simulink library "thc"  (R2021b)
settings: Solver=VariableStepAuto  StartTime=0.0  StopTime=10.0  RelTol=1e-3
undefined symbols (not defined in the file or in its folder): ATHC_APTCQA_X_C, ATHC_APTCQB_X_C, ATHC_dAy_X_C, ATHC_Qeq_X_kmh, ATHC_VbaseC_X_C, ATHC_VbaseC_Y_W, ATHC_VbaseD_X_C, ATHC_VbaseH_X_C, FALSE, KTHC_ACMaxMinT_sec, KTHC_aDeice_K, KTHC_AGSDefLv_K, KTHC_AGSLv1_K, KTHC_AGSLv2_K, KTHC_AGSLv3_K, KTHC_AGSLv4_K, KTHC_AGSLv5_K, KTHC_AirIntUpdateT_sec, KTHC_APTCOneZoneMax_W, KTHC_APTCPeriod_cnt, KTHC_APTCPWMEN_flg, KTHC_APTCQMaxC_W, KTHC_APTCQminC_W, KTHC_APTCQminD_W, KTHC_APTCQminRe1_W, KTHC_APTCQminRe_W, KTHC_APTCQoffT_cnt, KTHC_APTCQonT_cnt, KTHC_APTCRiLeMaxDff_W, KTHC_APTCRiLeMinDff_W, KTHC_BatInTempDef_C, KTHC_bDeice_K, KTHC_CompMaxDeice_rpm, KTHC_CompMinDeice_rpm, KTHC_CompSotxvOp_K, KTHC_CompSotxvOpLow_rpm, KTHC_CompSpdmax_rpm, KTHC_CompSpdmaxBC1_rpm, KTHC_CompSpdmaxBC_rpm, KTHC_CompSpdmid1_rpm, KTHC_CompSpdmid2_rpm, KTHC_CompSpdmid3_rpm, KTHC_CompSpdmid_rpm, KTHC_CompSpdmin_rpm, KTHC_DAPTCQ1_W, KTHC_DAPTCQ2_W, KTHC_DAPTCQ3_W, KTHC_DcChSetTemp_C, KTHC_DehumidityEN_flg, KTHC_DeiceCycTime_K, KTHC_DriveLevelWPTCBAH1_W, KTHC_DriveLevelWPTCBAH2_W, KTHC_DriveLevelWPTCBAH3_W, KTHC_DriveLevelWPTCBAH4_W, KTHC_DriveT1MinBAH_C, KTHC_DriveT2MaxBAH_C, KTHC_DriveT2MinBAH_C, KTHC_DriveT3MaxBAH_C, KTHC_DriveT3MinBAH_C, KTHC_DriveT4MaxBAH_C ... (+372)
libraries: simulink x140
(part 10 of 10)

== stateflow chart thc/THC/ThermalControl/THCM_Conctrl/APTC/APTCPWMControl1/Chart ==
  state APTC
    en:
    Wout=Win;
    du:
    Wout=Win;
  state APTCPWM
    (default) -> (junction 5) : {Tcnt=0;OnT=0;OffT=0;}
    APTCPWM -> (junction 5) [order 1]
    (junction 5) -> (junction 7) [order 1] : [Win==0]{Wout=0;}
    (junction 5) -> (junction 9) [order 2]
    (junction 7) -> (junction 11)
    (junction 9) -> (junction 11) [order 1] : [Win>Wmin]{Wout=Win;}
    (junction 9) -> (junction 54) [order 2]
    (junction 11) -> (junction 56)
    (junction 54) -> (junction 56) [order 1] : [Wout>Wmin]{Tcnt=0;Wout=0;....
        | OnT=Tp*Win/Wmin;OffT=Tp-OnT;}
    (junction 54) -> (junction 13) [order 2]
    (junction 56) -> (junction 15)
    (junction 13) -> (junction 15) [order 1] : [Wout>0&&Tcnt>=OnT]
        | {Tcnt=0;Wout=0;}
    (junction 13) -> (junction 17) [order 2]
    (junction 15) -> (junction 19)
    (junction 17) -> (junction 19) [order 1] : [Wout==0&&Tcnt>=OffT]
        | {Tcnt=0;Wout=Wmin;....
        | OnT=Tp*Win/Wmin;OffT=Tp-OnT;}
    (junction 17) -> (junction 26) [order 2]
    (junction 19) -> (junction 28)
    (junction 26) -> (junction 28)
    (junction 28) -> (junction 31) [order 2] : {Tcnt=Tcnt+1;}
    (junction 28) -> (junction 33) [order 1] : [Tcnt>Tp||(OnT==0&&OffT==0)]
        | {Tcnt=0;OnT=0;OffT=0;}
  (default) -> (junction 50)
  (junction 50) -> APTC [order 1] : [!KTHC_APTCPWMEN_flg]
  (junction 50) -> APTCPWM [order 2]
  APTCPWM -> APTC [order 1] : [!KTHC_APTCPWMEN_flg]
  APTC -> APTCPWM : [KTHC_APTCPWMEN_flg]
  data: OnT local uint16; OffT local uint16; Tcnt local uint16; Win input; Wout output uint16; Tp input uint16; Wmin input; KTHC_APTCPWMEN_flg input

== stateflow chart thc/THC/ThermalControl/THCM_Conctrl/APTC/APTCPWMControl2/Chart ==
  state APTC
    en:
    Wout=Win;
    du:
    Wout=Win;
  state APTCPWM
    (default) -> (junction 5) : {Tcnt=0;OnT=0;OffT=0;}
    APTCPWM -> (junction 5) [order 1]
    (junction 5) -> (junction 7) [order 1] : [Win==0]{Wout=0;}
    (junction 5) -> (junction 9) [order 2]
    (junction 7) -> (junction 11)
    (junction 9) -> (junction 11) [order 1] : [Win>Wmin]{Wout=Win;}
    (junction 9) -> (junction 54) [order 2]
    (junction 11) -> (junction 56)
    (junction 54) -> (junction 56) [order 1] : [Wout>Wmin]{Tcnt=0;Wout=0;....
        | OnT=Tp*Win/Wmin;OffT=Tp-OnT;}
    (junction 54) -> (junction 13) [order 2]
    (junction 56) -> (junction 15)
    (junction 13) -> (junction 15) [order 1] : [Wout>0&&Tcnt>=OnT]
        | {Tcnt=0;Wout=0;}
    (junction 13) -> (junction 17) [order 2]
    (junction 15) -> (junction 19)
    (junction 17) -> (junction 19) [order 1] : [Wout==0&&Tcnt>=OffT]
        | {Tcnt=0;Wout=Wmin;....
        | OnT=Tp*Win/Wmin;OffT=Tp-OnT;}
    (junction 17) -> (junction 26) [order 2]
    (junction 19) -> (junction 28)
    (junction 26) -> (junction 28)
    (junction 28) -> (junction 31) [order 2] : {Tcnt=Tcnt+1;}
    (junction 28) -> (junction 33) [order 1] : [Tcnt>Tp||(OnT==0&&OffT==0)]
        | {Tcnt=0;OnT=0;OffT=0;}
  (default) -> (junction 50)
  (junction 50) -> APTC [order 1] : [!KTHC_APTCPWMEN_flg]
  (junction 50) -> APTCPWM [order 2]
  APTCPWM -> APTC [order 1] : [!KTHC_APTCPWMEN_flg]
  APTC -> APTCPWM : [KTHC_APTCPWMEN_flg]
  data: OnT local uint16; OffT local uint16; Tcnt local uint16; Win input; Wout output uint16; Tp input uint16; Wmin input; KTHC_APTCPWMEN_flg input

== stateflow chart thc/THC/ThermalControl/THCM_Conctrl/BlowerCtrl/Chart ==
  state VGainCal
    (default) -> (junction 7)
    (junction 7) -> (junction 8) [order 1] : [VFull]
    (junction 7) -> (junction 10) [order 2] : {VGain=KTHC_VBRearClosed_K;}
    (junction 8) -> (junction 12) : {VGain=1;}
    (junction 10) -> (junction 12)
    (junction 12) -> (junction 15)
    VGainCal -> (junction 17) [order 1] : [VFull&&VGain<1]
    (junction 17) -> (junction 19) [order 1] : [VGain+KTHC_VGainStep_K<1]
    (junction 17) -> (junction 25) [order 2] : {VGain=1;}
    (junction 19) -> (junction 23) : {VGain=VGain+KTHC_VGainStep_K;}
    (junction 25) -> (junction 23)
    (junction 23) -> (junction 15)
    (junction 15) -> (junction 36)
    VGainCal -> (junction 21) [order 2] : [!VFull&&VGain>KTHC_VBRearClosed_K]
    (junction 21) -> (junction 28) [order 1] : [VGain-KTHC_VGainStep_K>KTHC_VBRearClosed_K]
    (junction 21) -> (junction 30) [order 2] : {VGain=KTHC_VBRearClosed_K;}
    (junction 28) -> (junction 32) : {VGain=VGain-KTHC_VGainStep_K;}
    (junction 30) -> (junction 32)
    (junction 32) -> (junction 36)
  data: VGain output single; VFull input boolean; KTHC_VBRearClosed_K input; KTHC_VGainStep_K input

== stateflow chart thc/THC/ThermalControl/THCM_Conctrl/Subsystem3/Chart ==
  state FWVSWReqDet [parallel]
    settings: executionOrder=2
    state StandBy
    (default) -> FWVSWReqDet.StandBy : {FWVSWReq=false;}
    FWVSWReqDet.StandBy -> FWVSWReqDet.StandBy : [AllStopReq]{FWVSWReq=true;}
  state EWP12Stop [parallel]
    settings: executionOrder=1
    state SpeedBalance
      state Stop
        en:EWP12Stop=true;
      state Wait
      (default) -> EWP12Stop.SpeedBalance.Stop
      EWP12Stop.SpeedBalance.Wait -> EWP12Stop.SpeedBalance.Stop : [after(EWPStopT,tick)]
    state NotBalance
      en:EWP12Stop=false;
    (default) -> EWP12Stop.SpeedBalance
    EWP12Stop.SpeedBalance -> EWP12Stop.NotBalance : [EWP1!=EWP2||....
        | hasChanged(EWP1)||....
        | hasChanged(EWP2)]
    EWP12Stop.NotBalance -> EWP12Stop.SpeedBalance.Wait : [EWP1==EWP2]
  state ValveControl [parallel]
    settings: executionOrder=4
    state StandBy
      en:
      TWVKeep=false;
      FWVKeep=false;
      EWPKeep=false;
      ex:
      TWVKeep=true;
      FWVKeep=true;
    state WaitEWPPartBallance
    state WaitEWPallStop
      ex:FWVSWReq=false;
      FWVKeep=false;
    state EWPKeep
      en:EWPKeep=true;
      TWVKeep=false;
      ex:EWPKeep=false;
    (default) -> ValveControl.StandBy
    ValveControl.StandBy -> WaitEWPPartBallance [order 2] : [PartStopReq]
    ValveControl.StandBy -> (junction 42) [order 1]
    WaitEWPPartBallance -> (junction 42) [order 2]
    (junction 42) -> WaitEWPallStop : [FWVSWReq]
    (junction 97) -> ValveControl.StandBy [order 2]
    WaitEWPPartBallance -> EWPKeep [order 1] : [EWP12Stop]
    (junction 97) -> WaitEWPallStop [order 1] : [FWVSWReq]
    EWPKeep -> (junction 97) : [after(ValueSWT,tick)]
    WaitEWPallStop -> EWPKeep : [EWPAllStop]
  state EWPAllStop [parallel]
    settings: executionOrder=3
    state SpeedBalance
      state Stop
        en:EWPAllStop=true;
      state Wait
      (default) -> EWPAllStop.SpeedBalance.Stop
      EWPAllStop.SpeedBalance.Wait -> EWPAllStop.SpeedBalance.Stop : [after(EWPStopT,tick)]
    state NotBalance
      en:EWPAllStop=false;
    (default) -> EWPAllStop.SpeedBalance
    EWPAllStop.SpeedBalance -> EWPAllStop.NotBalance : [EWP1!=EWP2||....
        | EWP2!=EWP3]
    EWPAllStop.NotBalance -> EWPAllStop.SpeedBalance.Wait : [EWP1==EWP2&&....
        | EWP2==EWP3]
  data: TWVKeep output boolean; FWVKeep output boolean; PartStopReq input boolean; AllStopReq input boolean; EWP1 input uint8; EWP2 input uint8; EWP3 input uint8; EWP12Stop local boolean; EWPAllStop local boolean; EWPStopT input uint8; ValueSWT input uint8; EWPKeep output boolean; FWVSWReq local boolean

== stateflow chart thc/THC/ThermalControl/AC1/Chart ==
  state Sync [parallel]
    settings: executionOrder=1
    state WaitForIVI
    state Release
    state Press
      state Wait
      state Over10sec
        en:ACForceOFF=!ACForceOFF;
      (default) -> Wait
      Wait -> Over10sec : [after(100,tick)]
    (default) -> WaitForIVI : {CCU_SyncSts=EEP_CCUSyncSts;ACForceOFF=EEP_ACForceOFF;}
    WaitForIVI -> Sync.Release : [VINP_CANMsgValidIVI2_flg]
    Sync.Release -> Sync.Release [order 3] : [SyncCancel]
        | {CCU_SyncSts=false;}
    Sync.Release -> Sync.Release [order 2] : [hasChanged(sigSetTempZon2Req_CMD)&&....
        | (sigSetTempZon2Req_CMD) != (sigSetTempZon1Req_CMD)]
        | {CCU_SyncSts=false;}
    Sync.Release -> Sync.Press [order 1] : [FCP_FrEvt_BtnSyncReq]
        | {CCU_SyncSts=!CCU_SyncSts;}
    Sync.Press -> Sync.Release [order 1] : [!FCP_FrEvt_BtnSyncReq]
    Sync.Press -> Sync.Press [order 2] : [SyncCancel]
        | {CCU_SyncSts=false;}
    Sync.Press -> Sync.Press [order 3] : [hasChanged(sigSetTempZon2Req_CMD)&&....
        | (sigSetTempZon2Req_CMD) != (sigSetTempZon1Req_CMD)]
        | {CCU_SyncSts=false;}
  state Recycle [parallel]
    settings: executionOrder=15
    state Manual
      state Outter
        en:sigRecircSt=false;
        state ACOFF
          en:FD_RecyAuto_Cmd=0;
        state ACON
          en:FD_RecyAuto_Cmd=4;
        (default) -> (junction 1044)
        (junction 1044) -> ACOFF [order 1] : [!CCU_ACLampSts&&....
            | (CabinMode==11&&....
            | ACSubMode==1)]
        (junction 1044) -> ACON [order 2]
        ACON -> ACOFF : [!CCU_ACLampSts&&....
            | (CabinMode==11&&ACSubMode==1)]
        ACOFF -> ACON : [CCU_ACLampSts||....
            | (CabinMode!=11||ACSubMode!=1)]
      state Inner
        en:sigRecircSt=true;
        FD_RecyAuto_Cmd=0;
      (default) -> (junction 920)
      (junction 920) -> (junction 922) [order 1] : [EEP_sigRecircSt]
      (junction 920) -> Outter [order 2]
      (junction 922) -> Inner
      Inner -> Outter [order 2] : eDefogRecycle
      Outter -> Inner : eRecycleBtn
      Inner -> Outter [order 1] : eRecycleBtn
      (junction 839) -> Outter [order 1] : [sigRecircSt]
      (junction 839) -> Inner [order 2]
    state Auto
      state SetLowT
        en:sigRecircSt=false;FD_RecyAuto_Cmd=4;
      state Normal
        state AutoInner
          en:
          sigRecircSt=true;
          note: 2 min
          state Refresh
            en:
            FD_RecyAuto_Cmd=4;
          state Hold
            en:
            FD_RecyAuto_Cmd=0;
          (default) -> Hold
          Refresh -> Hold : [after(KTHC_RecyChange_min*600,tick)]
          Hold -> Refresh : [KTHC_RefreshEN_flg&&...
              | after(KTHC_RecyHold_min*600,tick)]
        note: 30 min
        state AutoOutter
          en:sigRecircSt=false;
          state Dehumidity
            en:FD_RecyAuto_Cmd=KTHC_RecyOutterD_enum;
          state Normal
            state LV5
              en:FD_RecyAuto_Cmd=4;
            state LV4
              en:FD_RecyAuto_Cmd=3;
            state LV3
              en:FD_RecyAuto_Cmd=2;
            state LV2
              en:FD_RecyAuto_Cmd=1;
            (junction 713) -> LV5 [order 1] : [Tamb>KTHC_T4Mmaxamb_C]
            (junction 713) -> (junction 719) [order 2]
            LV5 -> LV4 : [Tamb<KTHC_T5Mminamb_C]
            LV4 -> LV5 [order 1] : [Tamb>KTHC_T4Mmaxamb_C]
            (junction 719) -> LV4 [order 1] : [Tamb>KTHC_T3Mmaxamb_C]
            (junction 719) -> (junction 725) [order 2]
            LV4 -> LV3 [order 2] : [Tamb<KTHC_T4Mminamb_C]
            LV3 -> LV4 [order 1] : [Tamb>KTHC_T3Mmaxamb_C]
            (junction 725) -> LV3 [order 1] : [Tamb>KTHC_T2Mmaxamb_C]
            (junction 725) -> (junction 730) [order 2]
            LV3 -> LV2 [order 2] : [Tamb<KTHC_T3Mminamb_C]
            LV2 -> LV3 : [Tamb>KTHC_T2Mmaxamb_C]
            (junction 730) -> LV2
          (default) -> (junction 1030)
          (junction 1030) -> Dehumidity [order 1] : [CabinMode<7]
          (junction 1030) -> (junction 1034) [order 2]
          Dehumidity -> (junction 1034) : [CabinMode>=7]
          (junction 1034) -> (junction 713)
          Recycle.Auto.Normal.AutoOutter.Normal -> Dehumidity : [CabinMode<7]
        (default) -> (junction 752)
        (junction 752) -> AutoInner [order 1] : [CabinMode==3||....
            | CabinMode==6||....
            | (CabinMode==11&&....
            | ACSubMode==1)]
        (junction 752) -> (junction 754) [order 2]
        AutoInner -> (junction 754) : [CabinMode!=3&&....
            | CabinMode!=6&&....
            | (CabinMode!=11||....
            | ACSubMode!=1)]
        (junction 754) -> AutoOutter
        AutoOutter -> AutoInner : [CabinMode==3||CabinMode==6||....
            | (CabinMode==11&&ACSubMode==1)]
      (default) -> (junction 1010)
      (junction 1010) -> (junction 1014) [order 1]
      (junction 1014) -> SetLowT : [CabinMode==3&&(ACSubMode==2||ACSubMode==6||ACSubMode==7)....
          | &&SetTempZon1St_CMD==170&&Tamb<KTHC_Trecymin_C]
      SetLowT -> Recycle.Auto.Normal : [CabinMode!=3||(ACSubMode!=2&&ACSubMode!=6&&ACSubMode!=7)||....
          | SetTempZon1St_CMD>170||Tamb>=KTHC_Trecymin_C]
      (junction 1010) -> Recycle.Auto.Normal [order 2]
      Recycle.Auto.Normal -> (junction 1014)
    (default) -> (junction 914)
    (junction 914) -> Recycle.Manual [order 1] : [EEP_ACModeMem!=2||!EEP_RecAutoFlg]
        | {RecAutoFlg=EEP_RecAutoFlg;}
    (junction 914) -> (junction 917) [order 2]
    Recycle.Auto -> (junction 839) [order 3] : eRecycleBtn
    Recycle.Auto -> Outter [order 2] : [!CCU_AutoLampSts&&!RecAutoFlg&&!sigRecircSt]
    Recycle.Auto -> Outter [order 1] : eDefogRecycle
    Recycle.Auto -> Inner [order 4] : [!CCU_AutoLampSts&&!RecAutoFlg]
    Recycle.Manual -> Recycle.Auto [order 2] : eACMaxRec
    Recycle.Manual -> Recycle.Auto [order 1] : [CCU_AutoLampSts&&RecAutoFlg]
    (junction 917) -> Recycle.Auto
  state RecycleSW [parallel]
    settings: executionOrder=16
    state Release
    state Press
      en:Recycle.eRecycleBtn;
      RecAutoFlg=false;
    (default) -> RecycleSW.Release
    RecycleSW.Release -> RecycleSW.Press : [sigRecircReq]
    RecycleSW.Press -> RecycleSW.Release : [!sigRecircReq]
  state PETMODE [parallel]
    settings: executionOrder=18
    state OFF
      en:PET=false;
    state ON
      en:PET=true;
    (default) -> PETMODE.OFF
    PETMODE.OFF -> PETMODE.ON : [(PwrSta>0&&PwrSta<=3&&(OFF_AC_MODE==1||OFF_AC_MODE==2||VINP_RemoteAutoReq_flg))||(ForceAuto&&PwrSta>3)]
    PETMODE.ON -> PETMODE.OFF : [(PwrSta==0||PwrSta>3||(OFF_AC_MODE!=1&&OFF_AC_MODE!=2&&!VINP_RemoteAutoReq_flg))&&(!ForceAuto||PwrSta<=3)]
  state ACBtn [parallel]
    settings: executionOrder=2
    state Initial
    state Release
    state Press
      en:AC.ACMode.eACBtn;
      WaterFill.eACBtn;
    (default) -> ACBtn.Initial
    ACBtn.Initial -> (junction 899) [order 2]
    (junction 899) -> ACBtn.Press
    ACBtn.Initial -> ACBtn.Release [order 1] : [EEP_ACModeMem!=1]
    ACBtn.Press -> ACBtn.Release : [!FCP_FrEvt_BtnACReq]
    ACBtn.Release -> ACBtn.Press : [FCP_FrEvt_BtnACReq]
  state ACAutoBtn [parallel]
    settings: executionOrder=3
    state Initial
    state Release
    state Press
      en:
      WaterFill.eACAutoBtn;
      RecAutoFlg=true;
    (default) -> ACAutoBtn.Initial
    ACAutoBtn.Initial -> (junction 904) [order 2] : {AC.ACMode.eACAutoBtn;}
    (junction 904) -> ACAutoBtn.Release
    ACAutoBtn.Initial -> ACAutoBtn.Release [order 1] : [EEP_ACModeMem!=2]
    ACAutoBtn.Release -> (junction 700) : [FCP_FrEvt_BtnAutoReq]
    (junction 700) -> ACAutoBtn.Press [order 1] : [CCU_AutoLampSts]{AC.ACMode.eAutoexit;}
    (junction 700) -> (junction 702) [order 2]
    (junction 702) -> ACAutoBtn.Press : {AC.ACMode.eACAutoBtn;}
    ACAutoBtn.Press -> ACAutoBtn.Release : [!FCP_FrEvt_BtnAutoReq]
  state ACMaxBtn [parallel]
    settings: executionOrder=4
    state Release
    state Press
      en:AC.ACMode.eACMaxBtn;
    (default) -> ACMaxBtn.Release
    ACMaxBtn.Release -> ACMaxBtn.Press : [FCP_FrEvt_BtnACMaxReq]
    ACMaxBtn.Press -> ACMaxBtn.Release : [!FCP_FrEvt_BtnACMaxReq]
  state ScreenBtn [parallel]
    settings: executionOrder=8
    state Release
    state Press
      en:AC.ACMode.eAutoexit;
    (default) -> ScreenBtn.Release
    ScreenBtn.Press -> ScreenBtn.Release : [!sigScreenReq]
    ScreenBtn.Release -> (junction 1060) : [sigScreenReq]{fdefog=false;}
    (junction 1060) -> ScreenBtn.Press [order 1] : [!Face&&!Foot&&Frost]
    (junction 1060) -> (junction 1061) [order 2]
    (junction 1061) -> ScreenBtn.Press : {Frost=!Frost;}
  state FaceBtn [parallel]
    settings: executionOrder=5
    state Press
      en:AC.ACMode.eAutoexit;
    state Release
    (default) -> FaceBtn.Release : {Face=EEP_Face;}
    FaceBtn.Press -> FaceBtn.Release : [!sigFaceReq]
    FaceBtn.Release -> (junction 183) : [sigFaceReq]{fdefog=false;}
    (junction 183) -> FaceBtn.Press [order 1] : [Face&&!Foot&&!Frost]
    (junction 183) -> (junction 185) [order 2]
    (junction 185) -> FaceBtn.Press : {Face=!Face;}
  state FootBtn [parallel]
    settings: executionOrder=6
    state Release
    state Press
      en:AC.ACMode.eAutoexit;
    (default) -> FootBtn.Release : {Foot=EEP_Foot;}
    FootBtn.Press -> FootBtn.Release : [!sigFootReq]
    FootBtn.Release -> (junction 189) : [sigFootReq]{fdefog=false;}
    (junction 189) -> FootBtn.Press [order 1] : [!Face&&Foot&&!Frost]
    (junction 189) -> (junction 197) [order 2]
    (junction 197) -> FootBtn.Press : {Foot=!Foot;}
  state Frost [parallel]
    settings: executionOrder=7
    state Press
      en:AC.ACMode.eAutoexit;
      ACModeMem=1;
    state Release
    (default) -> Frost.Release : {Frost=EEP_Frost;FaceM=EEP_FaceM;FootM=EEP_FootM;fdefog=EEP_fdefog;}
    Frost.Press -> Frost.Release : [!sigFrostReq]
    Frost.Release -> (junction 206) : [sigFrostReq]
    (junction 206) -> (junction 1208) [order 1] : [KTHC_ScreenUniq_flg&&!fdefog]
    (junction 206) -> (junction 1204) [order 2]
    (junction 1208) -> (junction 1206)
    (junction 1204) -> (junction 1206) [order 1] : [!KTHC_ScreenUniq_flg&&!Frost]
    (junction 1206) -> Frost.Press : {Frost=true;FaceM=Face;FootM=Foot;....
        | Face=false;Foot=false;fdefog=true;....
        | Recycle.eDefogRecycle;RecAutoFlg=false;}
    (junction 1204) -> (junction 200) [order 2]
    (junction 200) -> (junction 1212) [order 1] : [!Face&&!Foot]{Face=FaceM;Foot=FootM;fdefog=false;}
    (junction 1212) -> Frost.Press [order 1] : [!FaceM&&!FootM]{Frost=true;}
    (junction 200) -> (junction 769) [order 2]
    (junction 1212) -> (junction 1214) [order 2]
    (junction 1214) -> Frost.Press : {Frost=false;}
    (junction 769) -> Frost.Press : {Frost=false;fdefog=false;}
  state HMIWindDir [parallel]
    settings: executionOrder=9
    state StandBy
      ex:fdefog=0;
    (default) -> StandBy
    StandBy -> (junction 1100) [order 1] : [WindDirP]
    (junction 1100) -> (junction 1129) [order 1] : [sigWindDirZon1St==6]
        | {sigWindDirZon1StTemp=0;}
    (junction 1100) -> (junction 1127) [order 2]
    (junction 1129) -> (junction 1130)
    (junction 1127) -> (junction 1130) : {sigWindDirZon1StTemp=sigWindDirZon1St+1;}
    (junction 1130) -> (junction 1136)
    StandBy -> (junction 1133) [order 2] : [WindDirM]
    (junction 1133) -> (junction 1136) [order 1] : [sigWindDirZon1St==0]
        | {sigWindDirZon1StTemp=6;}
    (junction 1133) -> (junction 1138) [order 2]
    (junction 1136) -> (junction 1140)
    (junction 1138) -> (junction 1140) : {sigWindDirZon1StTemp=sigWindDirZon1St-1;}
    (junction 1140) -> (junction 1153)
    (junction 1153) -> StandBy [order 1] : [sigWindDirZon1StTemp==0]{Face=1;Foot=0;Frost=0;}
    (junction 1153) -> (junction 1156) [order 2]
    (junction 1156) -> StandBy [order 1] : [sigWindDirZon1StTemp==1]{Face=1;Foot=1;Frost=0;}
    (junction 1156) -> (junction 1159) [order 2]
    (junction 1159) -> StandBy [order 1] : [sigWindDirZon1StTemp==2]{Face=0;Foot=1;Frost=0;}
    (junction 1159) -> (junction 1162) [order 2]
    (junction 1162) -> StandBy [order 1] : [sigWindDirZon1StTemp==3]{Face=0;Foot=1;Frost=1;}
    (junction 1162) -> (junction 1165) [order 2]
    (junction 1165) -> StandBy [order 1] : [sigWindDirZon1StTemp==4]{Face=0;Foot=0;Frost=1;}
    (junction 1165) -> (junction 1168) [order 2]
    (junction 1168) -> StandBy [order 1] : [sigWindDirZon1StTemp==5]{Face=1;Foot=0;Frost=1;}
    (junction 1168) -> (junction 1171) [order 2]
    (junction 1171) -> StandBy : {Face=1;Foot=1;Frost=1;}
  state AC [parallel]
    settings: executionOrder=17
    state ACMode
      state ON
        state Max
          en:
          CCU_ACLampSts=true;
          CCU_AutoLampSts=false;
          CCU_ACMaxLampSts=true;
          sigAirIntenZon1St=9;
          CCU_SyncSts=true;
          Recycle.eACMaxRec;
          RecAutoFlg=true;
          state WaitMinT
          state WaitFinish
          (default) -> WaitMinT
          WaitMinT -> WaitFinish : [after(KTHC_ACMaxMinT_sec*10,tick)]
        state Manual
          en:
          CCU_ACLampSts=true;CCU_AutoLampSts=false;
          CCU_ACMaxLampSts=false;ACModeMem=1;
          RecAutoFlg=false;
          ACModeMem = 1;
          state Normal
            en:
            sigAirIntenZon1St=AirIntenZone1M;
            du:
            sigAirIntenZon1St=AirIntenZone1M;
          state DeFog
            en:
            sigAirIntenZon1St=9;
            ex:
            fdefog=false;
          (default) -> (junction 779)
          (junction 779) -> DeFog [order 2]
          (junction 779) -> AC.ACMode.ON.Manual.Normal [order 1] : [!fdefog]
          DeFog -> AC.ACMode.ON.Manual.Normal : [!fdefog]
          AC.ACMode.ON.Manual.Normal -> DeFog : [fdefog]
        state Auto
          en:
          CCU_ACLampSts=true;
          CCU_AutoLampSts=true;
          CCU_ACMaxLampSts=false;
          ACModeMem=2;
        WaitFinish -> (junction 851) : [MaxFinish||....
            | !CCU_SyncSts]
        Max -> AC.ACMode.ON.Manual [order 2] : eACMaxexit
        AC.ACMode.ON.Manual -> Max : eACMaxBtn
        Max -> (junction 850) [order 1] : eACMaxBtn
        AC.ACMode.ON.Auto -> Max [order 1] : eACMaxBtn
        (junction 850) -> (junction 851)
        (junction 851) -> (junction 49)
        (junction 49) -> AC.ACMode.ON.Manual [order 2]
        (junction 49) -> AC.ACMode.ON.Auto [order 1] : [ACModeMem==2]
        AC.ACMode.ON.Auto -> AC.ACMode.ON.Manual [order 2] : eAutoexit
        AC.ACMode.ON -> AC.ACMode.ON.Auto [order 1] : eACAutoBtn
        (default) -> (junction 943)
        (junction 943) -> AC.ACMode.ON.Manual [order 2]
        (junction 943) -> AC.ACMode.ON.Auto [order 1] : [ACModeMem == 2]
      state OFF
        en:
        CCU_ACLampSts=false;
        CCU_AutoLampSts=false;
        CCU_ACMaxLampSts=false;
        ACModeMem=0;
        sigAirIntenZon1St=AirIntenZone1M;
        du:
        sigAirIntenZon1St=AirIntenZone1M;
      (default) -> AC.ACMode.OFF
      AC.ACMode.OFF -> (junction 669) [order 4] : eACMaxBtn{ACModeMem=1;}
      (junction 669) -> Max [order 1] : [AirIntenZone1M!=1]
      (junction 669) -> (junction 671) [order 2]
      (junction 671) -> Max : {AirIntenZone1M=2;}
      AC.ACMode.ON -> AC.ACMode.OFF [order 1] : eACBtn
      AC.ACMode.OFF -> (junction 832) [order 2] : eACBtn
      (junction 832) -> (junction 833)
      AC.ACMode.OFF -> (junction 833) [order 1] : [fdefog]
      (junction 833) -> (junction 674)
      (junction 674) -> AC.ACMode.ON.Manual [order 1] : [AirIntenZone1M!=1]
      (junction 674) -> (junction 677) [order 2]
      (junction 677) -> AC.ACMode.ON.Manual : {AirIntenZone1M=2;}
      AC.ACMode.ON -> AC.ACMode.OFF [order 2] : [sigAirIntenZon1Req==1]
      (junction 683) -> AC.ACMode.ON.Auto [order 1] : [AirIntenZone1M!=1]
      AC.ACMode.OFF -> (junction 683) [order 3] : eACAutoBtn
      (junction 683) -> (junction 680) [order 2]
      (junction 680) -> AC.ACMode.ON.Auto : {AirIntenZone1M=2;}
      (junction 948) -> AC.ACMode.OFF [order 1] : [ACModeMem == 0]
      (junction 948) -> AC.ACMode.ON [order 2]
      (junction 947) -> (junction 948)
    state PET
      en:
      CCU_ACLampSts=true;
      CCU_AutoLampSts=true;
      CCU_ACMaxLampSts=false;
    (default) -> ACMode
    ACMode -> PET : [PET]
    PET -> (junction 947) : [!PET]
  state AutoWindDir [parallel]
    settings: executionOrder=14
    state Manmual
    state Standby
    (default) -> (junction 560)
    (junction 560) -> Manmual [order 1] : [!CCU_AutoLampSts]
    (junction 560) -> (junction 871) [order 2]
    Standby -> (junction 871) [order 3] : [hasChanged(VTHC_FootCold_flg)]
    (junction 871) -> (junction 578)
    Manmual -> (junction 578) : [CCU_AutoLampSts]
    Standby -> (junction 578) [order 1] : [after(KTHC_WindDirUpdateT_min*600,tick)||hasChanged(SetTempZon1St_CMD)]
    (junction 578) -> (junction 562)
    (junction 562) -> (junction 568) [order 1] : [Tamb<20]
    (junction 568) -> Standby [order 1] : [sigSetTempZon1St<Tincar||VTHC_FootCold_flg]....
        | {Face=KTHC_WDZ2Face_flg;Foot=KTHC_WDZ2Foot_flg;Frost=KTHC_WDZ2Frost_flg;}
    (junction 562) -> (junction 573) [order 2]
    (junction 568) -> (junction 570) [order 2]
    (junction 570) -> Standby : {Face=KTHC_WDZ1Face_flg;Foot=KTHC_WDZ1Foot_flg;Frost=KTHC_WDZ1Frost_flg;}
    (junction 575) -> Standby [order 1] : [Tincar-Tamb>KTHC_Tmidlevel_C]....
        | {Face=KTHC_WDZ5Face_flg;Foot=KTHC_WDZ5Foot_flg;Frost=KTHC_WDZ5Frost_flg;}
    (junction 573) -> (junction 575) [order 1] : [Tamb<25]
    (junction 573) -> (junction 581) [order 2]
    (junction 575) -> (junction 605) [order 2]
    (junction 605) -> Standby [order 1] : [sigSetTempZon1St<Tincar||VTHC_FootCold_flg]....
        | {Face=KTHC_WDZ3Face_flg;Foot=KTHC_WDZ3Foot_flg;Frost=KTHC_WDZ3Frost_flg;}
    (junction 605) -> (junction 608) [order 2]
    (junction 608) -> Standby : {Face=KTHC_WDZ4Face_flg;Foot=KTHC_WDZ4Foot_flg;Frost=KTHC_WDZ4Frost_flg;}
    (junction 624) -> Standby [order 1] : [sigSetTempZon1St<Tincar]....
        | {Face=KTHC_WDZ9Face_flg;Foot=KTHC_WDZ9Foot_flg;Frost=KTHC_WDZ9Frost_flg;}
    (junction 581) -> (junction 624) [order 1] : [Tincar-Tamb>KTHC_Thilevel2_C]
    (junction 581) -> (junction 583) [order 2]
    (junction 624) -> (junction 625) [order 2]
    (junction 625) -> Standby : {Face=KTHC_WDZ8Face_flg;Foot=KTHC_WDZ8Foot_flg;Frost=KTHC_WDZ8Frost_flg;}
    (junction 1051) -> (junction 625) [order 2]
    (junction 583) -> (junction 1051) [order 1] : [Tincar-Tamb>KTHC_Thilevel1_C]
    (junction 1051) -> Standby [order 1] : [sigSetTempZon1St<Tincar]....
        | {Face=KTHC_WDZ10Face_flg;Foot=KTHC_WDZ10Foot_flg;Frost=KTHC_WDZ10Frost_flg;}
    (junction 583) -> (junction 586) [order 2]
    (junction 586) -> Standby [order 1] : [sigSetTempZon1St>=Tincar]....
        | {Face=KTHC_WDZ7Face_flg;Foot=KTHC_WDZ7Foot_flg;Frost=KTHC_WDZ7Frost_flg;}
    (junction 586) -> (junction 589) [order 2]
    (junction 589) -> Standby : {Face=KTHC_WDZ6Face_flg;Foot=KTHC_WDZ6Foot_flg;Frost=KTHC_WDZ6Frost_flg;}
    Standby -> Manmual [order 2] : [!CCU_AutoLampSts]
  state WindDir [parallel]
    settings: executionOrder=10
    state Face
      en:sigWindDirZon1St=0;
    state Bilevel
      en:sigWindDirZon1St=1;
    state Foot
      en:sigWindDirZon1St=2;
    state FootandScreen
      en:sigWindDirZon1St=3;
    state Defog
      en:sigWindDirZon1St=4;
    state FaceandScreen
      en:sigWindDirZon1St=5;
    state AllOpen
      en:sigWindDirZon1St=6;
    state AllClose
      en:sigWindDirZon1St=7;
    (default) -> (junction 457)
    WindDir -> (junction 457) : [hasChanged(Face)||....
        | hasChanged(Foot)||....
        | hasChanged(Frost)]
    (junction 457) -> Face [order 1] : [Face&&!Foot&&!Frost]
    (junction 457) -> (junction 464) [order 2]
    (junction 464) -> Bilevel [order 1] : [Face&&Foot&&!Frost]
    (junction 464) -> (junction 467) [order 2]
    (junction 467) -> Foot [order 1] : [!Face&&Foot&&!Frost]
    (junction 467) -> (junction 472) [order 2]
    (junction 472) -> FootandScreen [order 1] : [!Face&&Foot&&Frost]
    (junction 472) -> (junction 476) [order 2]
    (junction 476) -> Defog [order 1] : [!Face&&!Foot&&Frost]
    (junction 476) -> (junction 480) [order 2]
    (junction 480) -> FaceandScreen [order 1] : [Face&&!Foot&&Frost]
    (junction 480) -> (junction 484) [order 2]
    (junction 484) -> AllOpen [order 1] : [Face&&Foot&&Frost]
    (junction 484) -> AllClose [order 2]
  state WaterFill [parallel]
    settings: executionOrder=11
    state Count1
    state OFF
      en:WaterFillReq=0;
      WFCnt=0;
    state Count
      en:WFCnt=WFCnt+1;
    state WaterFill2
      en:WaterFillReq=2;
    state WaterFill1
      en:WaterFillReq=1;
    (default) -> WaterFill.OFF
    WaterFill.OFF -> Count1 [order 2] : [FCP_FrEvt_BtnACReq]
    Count1 -> WaterFill.OFF [order 1] : [!FCP_FrEvt_BtnACReq]
    WaterFill.OFF -> Count [order 1] : eACAutoBtn....
        | [SetTempZon1St_CMD == 220 &&...
        |  SetTempZon2St_CMD == 310]
    Count -> WaterFill.OFF [order 3] : [SetTempZon1St_CMD != 220 ||...
        |  SetTempZon2St_CMD !=310 ||...
        | after(20,tick)]
    WaterFill1 -> WaterFill.OFF [order 1] : eACBtn
    (junction 1005) -> WaterFill.OFF : eACAutoBtn
    (junction 1002) -> WaterFill.OFF [order 1] : [after(36000,tick)||....
        | PwrSta==0||....
        | PwrSta==5]
    Count1 -> WaterFill2 [order 2] : [after(50,tick)]
    Count -> Count [order 2] : eACAutoBtn
    Count -> WaterFill1 [order 1] : [WFCnt>=3]
    (junction 1002) -> (junction 1005) [order 2]
    WaterFill2 -> (junction 1002)
    WaterFill1 -> (junction 1002) [order 2]
  state Manual [parallel]
    settings: executionOrder=12
    state Updated
      en:AC.ACMode.eAutoexit;
      CCU_AutoLampSts=false;
    state Auto
      state WaitForUpdate
      (default) -> (junction 953) : {FAutoFirst=true;}
      WaitForUpdate -> (junction 953) [order 2] : [after(2,tick)&&FAutoFirst]{FAutoFirst=false;}
      (junction 953) -> (junction 954)
      WaitForUpdate -> (junction 954) [order 3] : [FD_Blower_Cmd>AirIntHB||FD_Blower_Cmd<AirIntLB]
      (junction 954) -> (junction 955)
      WaitForUpdate -> (junction 955) [order 1] : [after(KTHC_AirIntUpdateT_sec*10,tick)]
      (junction 955) -> (junction 956)
      (junction 956) -> WaitForUpdate [order 1] : [FD_Blower_Cmd>=94]{sigAirIntenZon1St=9;AirIntLB=87.5;AirIntHB=100;}
      (junction 956) -> (junction 957) [order 2]
      (junction 957) -> WaitForUpdate [order 1] : [FD_Blower_Cmd>=82]{sigAirIntenZon1St=8;AirIntLB=75;AirIntHB=100;}
      (junction 957) -> (junction 958) [order 2]
      (junction 958) -> WaitForUpdate [order 1] : [FD_Blower_Cmd>=69]{sigAirIntenZon1St=7;AirIntLB=62.5;AirIntHB=87.5;}
      (junction 958) -> (junction 959) [order 2]
      (junction 959) -> WaitForUpdate [order 1] : [FD_Blower_Cmd>=56]{sigAirIntenZon1St=6;AirIntLB=50;AirIntHB=75;}
      (junction 959) -> (junction 960) [order 2]
      (junction 960) -> WaitForUpdate [order 1] : [FD_Blower_Cmd>=44]{sigAirIntenZon1St=5;AirIntLB=37.5;AirIntHB=62.5;}
      (junction 960) -> (junction 961) [order 2]
      (junction 961) -> WaitForUpdate [order 1] : [FD_Blower_Cmd>=32]{sigAirIntenZon1St=4;AirIntLB=25;AirIntHB=50;}
      (junction 961) -> (junction 962) [order 2]
      (junction 962) -> WaitForUpdate [order 1] : [FD_Blower_Cmd>=19]{sigAirIntenZon1St=3;AirIntLB=12.5;AirIntHB=37.5;}
      (junction 962) -> (junction 963) [order 2]
      (junction 963) -> WaitForUpdate : {sigAirIntenZon1St=2;;AirIntLB=0;AirIntHB=25;}
    (default) -> (junction 117) : {AirIntenZone1M=EEP_AirIntenZone1M;}
    (junction 117) -> Updated [order 2]
    (junction 117) -> Manual.Auto [order 1] : [CCU_AutoLampSts]
    Updated -> Manual.Auto : [CCU_AutoLampSts]
    Manual.Auto -> Updated : [!CCU_AutoLampSts]
    Manual -> (junction 1176) [order 2] : [AirIntP]
    (junction 1176) -> (junction 1178) [order 1] : [AirIntenZone1M<9]
        | {AirIntenZone1M=AirIntenZone1M+1;}
    (junction 1176) -> (junction 1180) [order 2]
    (junction 1178) -> (junction 1182)
    (junction 1180) -> (junction 1182)
    (junction 1182) -> (junction 1188)
    Manual -> (junction 1185) [order 3] : [AirIntM]
    (junction 1185) -> (junction 1188) [order 1] : [AirIntenZone1M>1]
        | {AirIntenZone1M=AirIntenZone1M-1;}
    (junction 1185) -> (junction 1191) [order 2]
    (junction 1188) -> (junction 1193)
    (junction 1191) -> (junction 1193)
    (junction 1193) -> (junction 817) : {fdefog=false;}
    Manual -> (junction 817) [order 1] : [hasChanged(sigAirIntenZon1Req)&&....
        | sigAirIntenZon1Req>0&&sigAirIntenZon1Req<10]....
        | {AirIntenZone1M=sigAirIntenZon1Req;fdefog=false;}
    (junction 817) -> Updated [order 1] : [CCU_ACMaxLampSts]....
        | {AC.ACMode.eACMaxexit;}
    (junction 817) -> (junction 819) [order 2]
    (junction 819) -> Updated
  state TFootUpdate [parallel]
    settings: executionOrder=13
    state Low
      en:
      VTHC_FootCold_flg=true;
    state High
      en:
      VTHC_FootCold_flg=false;
    (default) -> (junction 864)
    (junction 864) -> Low [order 1] : [T_Foot_min<KTHC_FootColdT_C]
    (junction 864) -> High [order 2]
    High -> Low : [T_Foot_min<KTHC_FootColdT_C]
    Low -> High : [T_Foot_min>KTHC_FootColdT_C+KTHC_FootColdTdelta_C]
  data: FCP_FrEvt_BtnACMaxReq input; FCP_FrEvt_BtnACReq input; FCP_FrEvt_BtnAutoReq input; FCP_FrEvt_BtnSyncReq input; FD_Blower_Cmd input; Tamb input; Tincar input; sigAirIntenZon1Req input; sigRecircReq input; CCU_ACLampSts output boolean; CCU_ACMaxLampSts output boolean; CCU_SyncSts output; sigAirIntenZon1St output; sigWindDirZon1St output; CCU_AutoLampSts output boolean; sigRecircSt output =0; sigFaceReq input; sigFootReq input; sigFrostReq input; sigSetTempZon1St input; SetTempZon1St_CMD input; SetTempZon2St_CMD input; PwrSta input; sigSetTempZon2Req_CMD input; sigSetTempZon1Req_CMD input; WaterFillReq output uint8; WFCnt local uint8; Frost output boolean; ACForceOFF output; KTHC_WindDirUpdateT_min input; KTHC_AirIntUpdateT_sec input; OFF_AC_MODE input; PET output boolean; FD_RecyAuto_Cmd output; KTHC_T2Mmaxamb_C input; KTHC_T3Mmaxamb_C input; KTHC_T4Mmaxamb_C input; KTHC_T3Mminamb_C input; KTHC_T4Mminamb_C input; KTHC_T5Mminamb_C input; KTHC_RecyHold_min input; KTHC_RecyChange_min input; KTHC_Tmidlevel_C input; KTHC_Thilevel1_C input; KTHC_Thilevel2_C input; CabinMode input; KTHC_WDZ1Face_flg input boolean; KTHC_WDZ1Foot_flg input boolean; KTHC_WDZ1Frost_flg input boolean; KTHC_WDZ2Face_flg input boolean; KTHC_WDZ2Foot_flg input boolean; KTHC_WDZ2Frost_flg input boolean; KTHC_WDZ3Face_flg input boolean; KTHC_WDZ3Foot_flg input boolean; KTHC_WDZ3Frost_flg input boolean; KTHC_WDZ4Face_flg input boolean; KTHC_WDZ4Foot_flg input boolean; KTHC_WDZ4Frost_flg input boolean; KTHC_WDZ5Face_flg input boolean; KTHC_WDZ5Foot_flg input boolean; KTHC_WDZ5Frost_flg input boolean; KTHC_WDZ6Face_flg input boolean; KTHC_WDZ6Foot_flg input boolean; KTHC_WDZ6Frost_flg input boolean; KTHC_WDZ7Face_flg input boolean; KTHC_WDZ7Foot_flg input boolean; KTHC_WDZ7Frost_flg input boolean; KTHC_WDZ8Face_flg input boolean; KTHC_WDZ8Foot_flg input boolean; KTHC_WDZ8Frost_flg input boolean; KTHC_WDZ9Face_flg input boolean; KTHC_WDZ9Foot_flg input boolean; KTHC_WDZ9Frost_flg input boolean; KTHC_WDZ10Face_flg input; KTHC_WDZ10Foot_flg input; KTHC_WDZ10Frost_flg input; ForceAuto input; KTHC_RefreshEN_flg input boolean; MaxFinish input; T_Foot_min input; KTHC_FootColdT_C input; KTHC_FootColdTdelta_C input; VTHC_FootCold_flg local boolean; KTHC_ACMaxMinT_sec input; FAutoFirst local boolean; ACModeMem output; EEP_ACModeMem input; EEP_Face input; EEP_Foot input; EEP_Frost input; EEP_FaceM input; EEP_FootM input; FaceM output boolean; FootM output boolean; Face output boolean; Foot output boolean; EEP_CCUSyncSts input; EEP_ACForceOFF input; EEP_sigRecircSt input; EEP_RecAutoFlg input; EEP_AirIntenZone1M input; EEP_fdefog input; fdefog output boolean; RecAutoFlg output boolean; AirIntenZone1M output; VINP_CANMsgValidIVI2_flg input; VINP_RemoteAutoReq_flg input; AirIntHB local double; AirIntLB local double; KTHC_Trecymin_C input; ACSubMode input; KTHC_RecyOutterD_enum input; SyncCancel input; WindDirP input; WindDirM input; AirIntP input; AirIntM input; sigWindDirZon1StTemp local uint8; sigScreenReq input; KTHC_ScreenUniq_flg input boolean
  events: eRecycleBtn local FUNCTION_CALL_EVENT; eDefogRecycle local FUNCTION_CALL_EVENT; eACMaxRec local FUNCTION_CALL_EVENT; eACBtn local FUNCTION_CALL_EVENT; eACMaxBtn local FUNCTION_CALL_EVENT; eACAutoBtn local FUNCTION_CALL_EVENT; eAutoexit local FUNCTION_CALL_EVENT; eACMaxexit local FUNCTION_CALL_EVENT; eACAutoBtn local FUNCTION_CALL_EVENT; eACBtn local FUNCTION_CALL_EVENT

== stateflow chart thc/THC/ThermalControl/AC1/Subsystem/Chart ==
  state MotorInitial
    state OFF
      en:FGSLearn=0;
      FGSEnable=TRUE;
    state SelfLearn
      state Initial
      state OFF
        en:FGSLearn=0x5A;
      state Ready
        en:FGSLearn=0;
        state WaitForChagned
          en:FGSEnable=FALSE;
        state Changed
          en:FGSEnable=TRUE;
        (default) -> WaitForChagned
        Ready -> WaitForChagned : [hasChanged(IVI_FGSCh_Cmd)]
        WaitForChagned -> Changed : [FGS_AirInt_Sta==0]
      Initial -> MotorInitial.SelfLearn.OFF [order 2] : [after(10,tick)]
      MotorInitial.SelfLearn.OFF -> Ready : [FGS_MotorInit_Sta==1]
      Initial -> Ready [order 1] : [FGS_MotorInit_Sta==3]
    (default) -> MotorInitial.OFF
    MotorInitial.OFF -> Initial : [PwrSta>3]
    SelfLearn -> MotorInitial.OFF : [PwrSta<=3]
  data: FGS_MotorInit_Sta input; PwrSta input; FGSLearn output uint8; IVI_FGSCh_Cmd input; FGS_AirInt_Sta input; FGSEnable output boolean; TRUE parameter; FALSE parameter

== stateflow chart thc/THC/ThermalControl/THCM_Conctrl/Subsystem/Chart ==
  state ForceCompOFF
    en:FCompOFF=True;
    Keep=True;
    EXVOpen=1;
  state StandBy
    en:FCompOFF=False;
    Keep=False;
    EXVOpen=0;
  state ForceCompOFF3
    en:
    Keep=False;
    EXVOpen=0;
  note: 2 sec
  note: 5 sec
  note: 5 sec
  state ForceCompOFF2
    en:
    Keep=False;
    EXVOpen=0;
  state ForceCompOFF1
    en:
    Keep=True;
    EXVOpen=2;
  note: 10 sec
  (default) -> StandBy
  StandBy -> (junction 26) : [SOV1C!=SOV1CBuf||SOV2C!=SOV2CBuf||SOV3C!=SOV3CBuf]
  (junction 26) -> ForceCompOFF [order 2]
  (junction 26) -> ForceCompOFF3 [order 1] : [Comp==0]{FCompOFF=True;}
  ForceCompOFF -> ForceCompOFF1 : [after(KTHC_PBlaceTime1_K,tick)]
  ForceCompOFF3 -> StandBy : [after(KTHC_PBlaceTime4_K,tick)]
  ForceCompOFF2 -> StandBy : [after(KTHC_PBlaceTime3_K,tick)]
  ForceCompOFF1 -> ForceCompOFF2 : [after(KTHC_PBlaceTime2_K,tick)]
  data: FCompOFF output boolean; SOV1C input; SOV1CBuf input; SOV2C input; SOV2CBuf input; SOV3C input; SOV3CBuf input; Keep output boolean; True constant boolean =boolean(1); False constant boolean =boolean(0); Comp input; KTHC_PBlaceTime1_K input; KTHC_PBlaceTime2_K input; KTHC_PBlaceTime3_K input; KTHC_PBlaceTime4_K input; EXVOpenflg local boolean; EXVOpen output uint8
